simulink model "comVisualization"  (Simulink 8.4)
settings: Solver=FixedStepDiscrete  StartTime=0.0  StopTime=inf  FixedStep=0.010  RelTol=1e-3
InitFcn:
  | Init;
  | visualizerParameters;
values from neighbouring files (symbols this model uses):
  figureHandle = figure    [visualizerParameters.m]
  footLength = 0.15    [visualizerParameters.m]
  footWidth = 0.08    [visualizerParameters.m]
  l_ankle_pitch = 18    [visualizerParameters.m]
  l_ankle_roll = 19    [visualizerParameters.m]
  r_ankle_pitch = 24    [visualizerParameters.m]
  r_ankle_roll = 25    [visualizerParameters.m]
  Ts = 0.006    [Init.m]
libraries: WBCLibrary x9
settings Model: Creator=jorhabib  LastModifiedBy=pucci
settings DataIOCC: SignalLoggingSaveFormat=Dataset
settings OptimizationCC: ExpressionDepthLimit=128
settings DebuggingCC: UnderspecifiedInitializationDetection=Simplified  MergeDetectMultiDrivingBlocksExec=error  FcnCallInpInsideContextMsg=EnableAllAsError  StateNameClashWarn=none
settings GRTTargetCC: CombineOutputUpdateFcns=on  GRTInterface=off

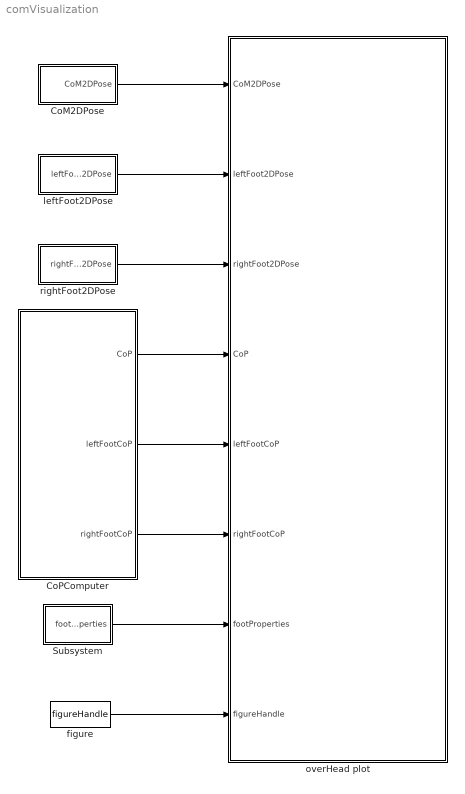
== system comVisualization ==
  CoM2DPose : Subsystem
  CoPComputer : Subsystem
  Subsystem : Subsystem
  figure : Constant  Value=figureHandle
  leftFoot2DPose : Subsystem
  overHead plot : MATLAB Function  TreatAsAtomicUnit=on
  rightFoot2DPose : Subsystem
  wires:
  CoM2DPose/1(CoM2DPose) -> overHead plot/1(CoM2DPose)
  CoPComputer/3(rightFootCoP) -> overHead plot/6(rightFootCoP)
  CoPComputer/2(leftFootCoP) -> overHead plot/5(leftFootCoP)
  CoPComputer/1(CoP) -> overHead plot/4(CoP)
  rightFoot2DPose/1(rightFoot2DPose) -> overHead plot/3(rightFoot2DPose)
  leftFoot2DPose/1(leftFoot2DPose) -> overHead plot/2(leftFoot2DPose)
  figure/1 -> overHead plot/8(figureHandle)
  Subsystem/1(footProperties) -> overHead plot/7(footProperties)

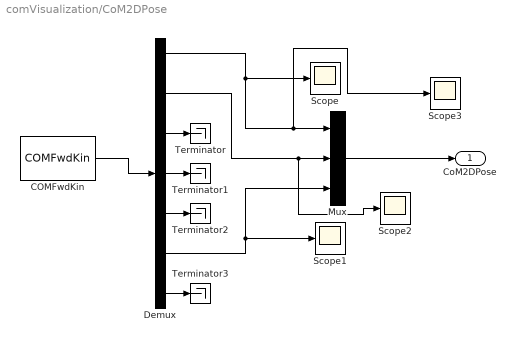
== system comVisualization/CoM2DPose ==
  "COMFwdKin " : WBCLibrary/wholeBodyModel/Forward Kinematics/COMFwdKin   robotName=robotName  localName=localName
  Demux : Demux  Outputs=7
  Mux : Mux  Inputs=3
  Scope{,1..3} (4 alike) : Scope
      Scope1 settings: SaveName=ScopeData5
      Scope2 settings: SaveName=ScopeData6
      Scope3 settings: SaveName=ScopeData7
  Terminator{,1..3} (4 alike) : Terminator
  CoM2DPose : Outport
  wires:
  Demux/3 -> Terminator/1
  Demux/2 -> Scope2/1, Mux/2
  "COMFwdKin "/1 -> Demux/1
  Demux/4 -> Terminator1/1
  Demux/5 -> Terminator2/1
  Mux/1 -> CoM2DPose/1
  Demux/6 -> Mux/3, Scope1/1
  Demux/1 -> Scope/1, Scope3/1, Mux/1
  Demux/7 -> Terminator3/1

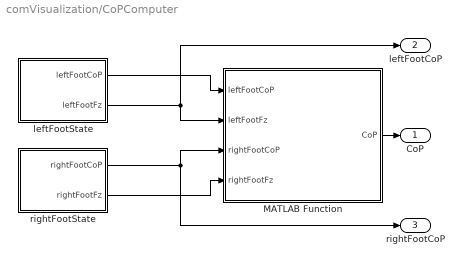
== system comVisualization/CoPComputer ==
  MATLAB Function : MATLAB Function  TreatAsAtomicUnit=on
  leftFootState : Subsystem
  rightFootState : Subsystem
  CoP : Outport
  leftFootCoP : Outport  Port=2
  rightFootCoP : Outport  Port=3
  wires:
  rightFootState/1(rightFootCoP) -> rightFootCoP/1, MATLAB Function/3(rightFootCoP)
  leftFootState/1(leftFootCoP) -> MATLAB Function/1(leftFootCoP)
  leftFootState/2(leftFootFz) -> leftFootCoP/1, MATLAB Function/2(leftFootFz)
  rightFootState/2(rightFootFz) -> MATLAB Function/4(rightFootFz)
  MATLAB Function/1(CoP) -> CoP/1

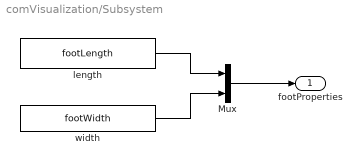
== system comVisualization/Subsystem ==
  Mux : Mux  Inputs=2
  length : Constant  Value=footLength
  width : Constant  Value=footWidth
  footProperties : Outport
  wires:
  length/1 -> Mux/1
  Mux/1 -> footProperties/1
  width/1 -> Mux/2

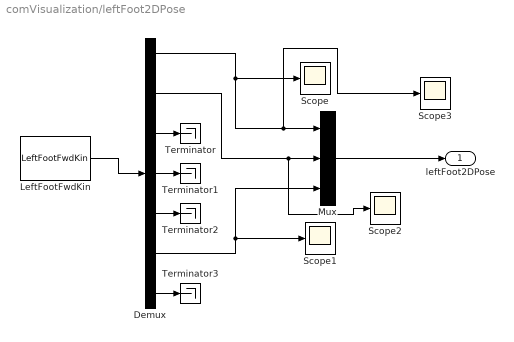
== system comVisualization/leftFoot2DPose ==
  Demux : Demux  Outputs=7
  LeftFootFwdKin : WBCLibrary/wholeBodyModel/Forward Kinematics/LeftFootFwdKin  robotName=robotName  localName=localName
      link override Input Param. for forwardKinematics and  computeJacobians 4: Value=zeros(ROBOT_DOF+6,1)
  Mux : Mux  Inputs=3
  Scope{,1..3} (4 alike) : Scope
      Scope1 settings: SaveName=ScopeData2
      Scope2 settings: SaveName=ScopeData3
      Scope3 settings: SaveName=ScopeData4
  Terminator{,1..3} (4 alike) : Terminator
  leftFoot2DPose : Outport
  wires:
  Demux/3 -> Terminator/1
  Demux/2 -> Scope2/1, Mux/2
  LeftFootFwdKin/1 -> Demux/1
  Demux/4 -> Terminator1/1
  Demux/5 -> Terminator2/1
  Mux/1 -> leftFoot2DPose/1
  Demux/6 -> Mux/3, Scope1/1
  Demux/1 -> Scope/1, Scope3/1, Mux/1
  Demux/7 -> Terminator3/1

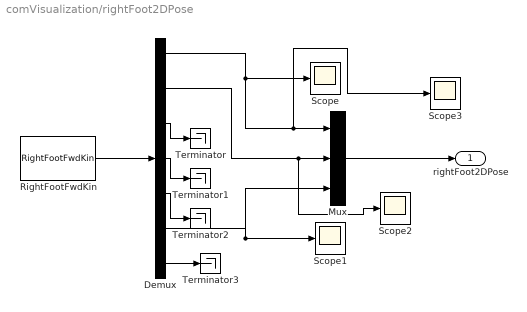
== system comVisualization/rightFoot2DPose ==
  Demux : Demux  Outputs=7
  Mux : Mux  Inputs=3
  RightFootFwdKin : WBCLibrary/wholeBodyModel/Forward Kinematics/RightFootFwdKin  robotName=robotName  localName=localName
  Scope{,1..3} (4 alike) : Scope
      Scope1 settings: SaveName=ScopeData2
      Scope2 settings: SaveName=ScopeData3
      Scope3 settings: SaveName=ScopeData4
  Terminator{,1..3} (4 alike) : Terminator
  rightFoot2DPose : Outport
  wires:
  Demux/3 -> Terminator/1
  Demux/2 -> Scope2/1, Mux/2
  RightFootFwdKin/1 -> Demux/1
  Demux/4 -> Terminator1/1
  Demux/5 -> Terminator2/1
  Mux/1 -> rightFoot2DPose/1
  Demux/6 -> Mux/3, Scope1/1
  Demux/1 -> Scope/1, Scope3/1, Mux/1
  Demux/7 -> Terminator3/1

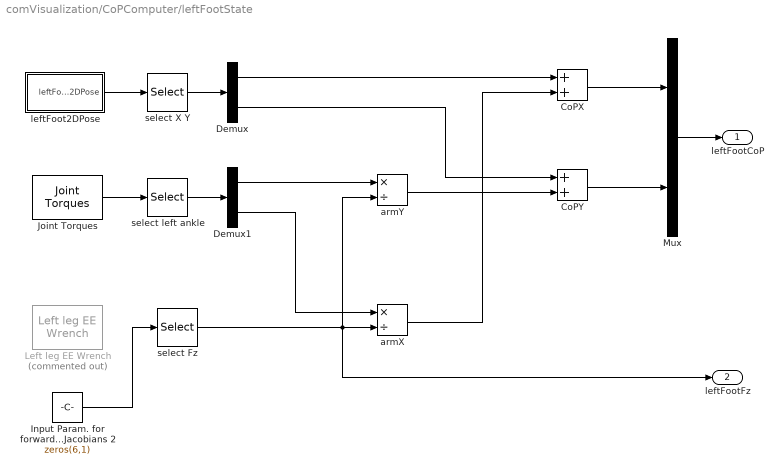
== system comVisualization/CoPComputer/leftFootState ==
  CoPX : Sum
  CoPY : Sum
  Demux : Demux  Outputs=2
  Demux1 : Demux  Outputs=2
  Input Param. for forwardKinematics and  computeJacobians 2 : Constant  Value=zeros(6,1)  OutDataTypeStr=double  SampleTime=Ts
  Joint Torques : WBCLibrary/wholeBodyStates/Joint Torques  robotName=robotName  localName=localName
  Left leg EE Wrench : WBCLibrary/wholeBodyStates/Left leg EE Wrench  Commented=on  robotName=robotName  localName=localName
  Mux : Mux  Inputs=2
  armX : Product  Inputs=*/
  armY : Product  Inputs=*/
  leftFoot2DPose : Subsystem
  select Fz : Selector  InputPortWidth=6  Indices=[3]
  select X Y : Selector  InputPortWidth=3  Indices=[1, 2]
  select left ankle : Selector  InputPortWidth=25  Indices=[l_ankle_pitch, l_ankle_roll]
  leftFootCoP : Outport
  leftFootFz : Outport  Port=2
  wires:
  select left ankle/1 -> Demux1/1
  CoPY/1 -> Mux/2
  CoPX/1 -> Mux/1
  armY/1 -> CoPY/2
  Mux/1 -> leftFootCoP/1
  Demux1/2 -> armX/1
  Demux/2 -> CoPY/1
  Demux/1 -> CoPX/1
  Joint Torques/1 -> select left ankle/1
  armX/1 -> CoPX/2
  Demux1/1 -> armY/1
  select X Y/1 -> Demux/1
  leftFoot2DPose/1(leftFoot2DPose) -> select X Y/1
  select Fz/1 -> leftFootFz/1, armX/2, armY/2
  Input Param. for forwardKinematics and  computeJacobians 2/1 -> select Fz/1

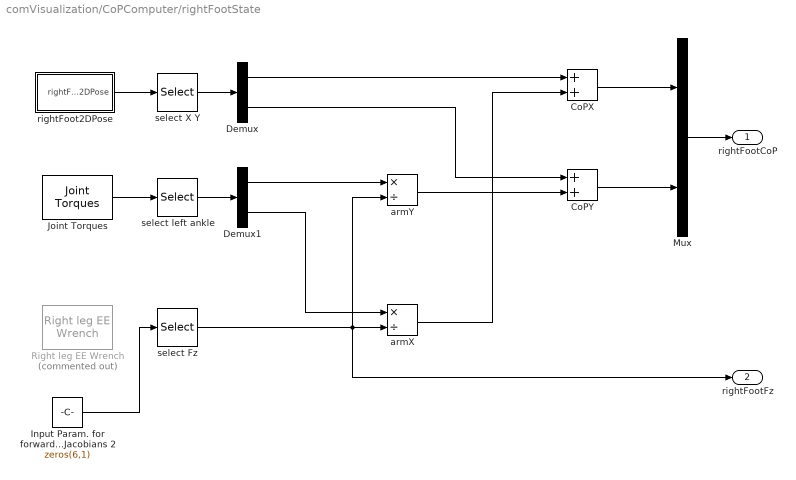
== system comVisualization/CoPComputer/rightFootState ==
  CoPX : Sum
  CoPY : Sum
  Demux : Demux  Outputs=2
  Demux1 : Demux  Outputs=2
  Input Param. for forwardKinematics and  computeJacobians 2 : Constant  Value=zeros(6,1)  OutDataTypeStr=double  SampleTime=Ts
  Joint Torques : WBCLibrary/wholeBodyStates/Joint Torques  robotName=robotName  localName=localName
  Mux : Mux  Inputs=2
  Right leg EE Wrench : WBCLibrary/wholeBodyStates/Right leg EE Wrench  Commented=on  robotName=robotName  localName=localName
  armX : Product  Inputs=*/
  armY : Product  Inputs=*/
  rightFoot2DPose : Subsystem
  select Fz : Selector  InputPortWidth=6  Indices=[3]
  select X Y : Selector  InputPortWidth=3  Indices=[1, 2]
  select left ankle : Selector  InputPortWidth=25  Indices=[r_ankle_pitch, r_ankle_roll]
  rightFootCoP : Outport
  rightFootFz : Outport  Port=2
  wires:
  select left ankle/1 -> Demux1/1
  CoPY/1 -> Mux/2
  CoPX/1 -> Mux/1
  armY/1 -> CoPY/2
  Mux/1 -> rightFootCoP/1
  Demux1/2 -> armX/1
  Demux/2 -> CoPY/1
  Demux/1 -> CoPX/1
  Joint Torques/1 -> select left ankle/1
  armX/1 -> CoPX/2
  Demux1/1 -> armY/1
  select X Y/1 -> Demux/1
  rightFoot2DPose/1(rightFoot2DPose) -> select X Y/1
  select Fz/1 -> rightFootFz/1, armX/2, armY/2
  Input Param. for forwardKinematics and  computeJacobians 2/1 -> select Fz/1

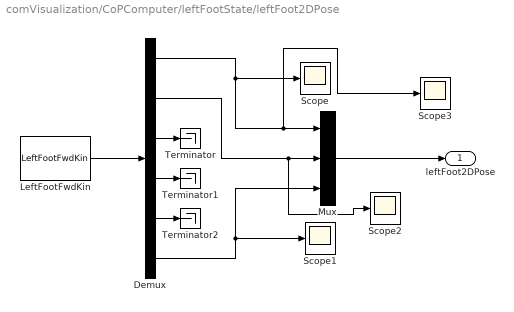
== system comVisualization/CoPComputer/leftFootState/leftFoot2DPose ==
  Demux : Demux  Outputs=6
  LeftFootFwdKin : WBCLibrary/wholeBodyModel/Forward Kinematics/LeftFootFwdKin  robotName=robotName  localName=localName
      link override Input Param. for forwardKinematics and  computeJacobians 4: Value=zeros(ROBOT_DOF+6,1)
  Mux : Mux  Inputs=3
  Scope{,1..3} (4 alike) : Scope
      Scope1 settings: SaveName=ScopeData2
      Scope2 settings: SaveName=ScopeData3
      Scope3 settings: SaveName=ScopeData4
  Terminator : Terminator
  Terminator1 : Terminator
  Terminator2 : Terminator
  leftFoot2DPose : Outport
  wires:
  Demux/3 -> Terminator/1
  Demux/2 -> Scope2/1, Mux/2
  LeftFootFwdKin/1 -> Demux/1
  Demux/4 -> Terminator1/1
  Demux/5 -> Terminator2/1
  Mux/1 -> leftFoot2DPose/1
  Demux/6 -> Mux/3, Scope1/1
  Demux/1 -> Scope/1, Scope3/1, Mux/1

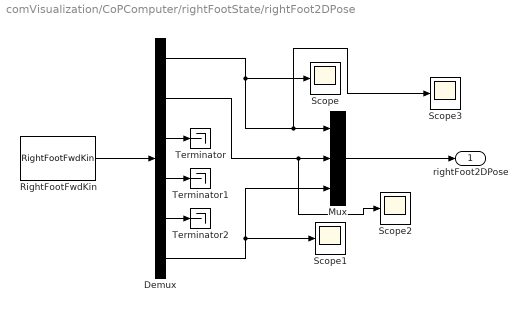
== system comVisualization/CoPComputer/rightFootState/rightFoot2DPose ==
  Demux : Demux  Outputs=6
  Mux : Mux  Inputs=3
  RightFootFwdKin : WBCLibrary/wholeBodyModel/Forward Kinematics/RightFootFwdKin  robotName=robotName  localName=localName
  Scope{,1..3} (4 alike) : Scope
      Scope1 settings: SaveName=ScopeData2
      Scope2 settings: SaveName=ScopeData3
      Scope3 settings: SaveName=ScopeData4
  Terminator : Terminator
  Terminator1 : Terminator
  Terminator2 : Terminator
  rightFoot2DPose : Outport
  wires:
  Demux/3 -> Terminator/1
  Demux/2 -> Scope2/1, Mux/2
  RightFootFwdKin/1 -> Demux/1
  Demux/4 -> Terminator1/1
  Demux/5 -> Terminator2/1
  Mux/1 -> rightFoot2DPose/1
  Demux/6 -> Mux/3, Scope1/1
  Demux/1 -> Scope/1, Scope3/1, Mux/1

== matlab function CoPComputer/MATLAB Function ==
  data: leftFootCoP input double; leftFootFz input double; CoP output double; rightFootCoP input double; rightFootFz input double
function CoP = fcn(leftFootCoP, leftFootFz, rightFootCoP, rightFootFz)
leftFootCoPX = leftFootCoP(1);
leftFootCoPY = leftFootCoP(2);
rightFootCoPX = rightFootCoP(1);
rightFootCoPY = rightFootCoP(2);
totFz = leftFootFz + rightFootFz;

CoPX = (leftFootCoPX * leftFootFz + rightFootCoPX * rightFootFz) / totFz; 
CoPY = (leftFootCoPY * leftFootFz + rightFootCoPY * rightFootFz) / totFz;

CoP = [CoPX, CoPY];

== matlab function overHead plot ==
  data: CoM2DPose input double; leftFoot2DPose input double; rightFoot2DPose input double; CoP input double; leftFootCoP input double; rightFootCoP input double; footProperties input double; figureHandle input double
function fcn(CoM2DPose, leftFoot2DPose, rightFoot2DPose, CoP, leftFootCoP, rightFootCoP, footProperties, figureHandle)
% constants
LEFT_FOOT_COLOR = 'r';
RIGHT_FOOT_COLOR = 'g';
CoM_COLOR = 'k';
CoP_COLOR = 'b';
FOOT_SCALE_FACTOR = 3;
CIRCLE_RADIUS = 4;

footLength = footProperties(1);
footWidth = footProperties(2);

leftFootCentroid = [leftFoot2DPose(1), leftFoot2DPose(2)];
leftFootYaw = 0.0; %leftFoot2DPose(3);
[leftX, leftY] = computeFourFootPolygonVertices(leftFootCentroid, leftFootYaw, footLength, footWidth);

rightFootCentroid = [rightFoot2DPose(1), rightFoot2DPose(2)];
rightFootYaw = 0.0; %rightFoot2DPose(3);
[rightX, rightY] = computeFourFootPolygonVertices(rightFootCentroid, rightFootYaw, footLength, footWidth);

prepareFigure(figureHandle, CoM2DPose, footLength, FOOT_SCALE_FACTOR);
drawCircle(CoM2DPose, CIRCLE_RADIUS, CoM_COLOR, figureHandle)
plotFootPolygon(leftX, leftY, LEFT_FOOT_COLOR, figureHandle);
plotFootPolygon(rightX, rightY, RIGHT_FOOT_COLOR, figureHandle);

function [x, y] = computeFourFootPolygonVertices(centroid, footYaw, footLength, footWidth)
NUMBER_OF_VERTICES = 4;

centroidX = centroid(1);
centroidY = centroid(2);
halfFootLength = footLength/2;
halfFootWidth = footWidth/2;
x = zeros(NUMBER_OF_VERTICES);
y = zeros(NUMBER_OF_VERTICES);

tempX = centroidX + halfFootLength;
tempY = centroidY + halfFootWidth;
[rotX, rotY] = rotate2DVector(tempX, tempY, footYaw);
x(1) = rotX;
y(1) = rotY;

tempX = centroidX - halfFootLength;
tempY = centroidY + halfFootWidth;
[rotX, rotY] = rotate2DVector(tempX, tempY, footYaw);
x(2) = rotX;
y(2) = rotY;

tempX = centroidX - halfFootLength;
tempY = centroidY - halfFootWidth;
[rotX, rotY] = rotate2DVector(tempX, tempY, footYaw);
x(3) = rotX;
y(3) = rotY;

tempX = centroidX + halfFootLength;
tempY = centroidY - halfFootWidth;
[rotX, rotY] = rotate2DVector(tempX, tempY, footYaw);
x(4) = rotX;
y(4) = rotY;

function plotFootPolygon(x, y, color, figureHandle)
numberOfVertices = length(x);

for i = 1 : numberOfVertices
    if i < numberOfVertices
        drawLine([x(i),y(i)],[x(i+1), y(i+1)], color, figureHandle);
    else
        drawLine([x(i),y(i)],[x(1), y(1)], color, figureHandle);
    end
end

function [] = drawLine(p1, p2, color, figureHandle)
theta = atan2( p2(2) - p1(2), p2(1) - p1(1));
r = sqrt( (p2(1) - p1(1))^2 + (p2(2) - p1(2))^2);

line = linspace(0,r,10);
x = p1(1) + line*cos(theta);
y = p1(2) + line*sin(theta);

figure(figureHandle);
plot(x, y, color)
drawnow;
hold on

function [] = drawCircle(position, radius, color, figureHandle)
x = position(1);
y = position(2);

figure(figureHandle);
plot(x, y, 'Color', color, 'Marker', 'o', 'MarkerSize', radius)
drawnow;
hold on

function [newX,newY] = rotate2DVector(x, y, angle)
newX = x * cos(angle) - y * sin(angle);
newY = x * sin(angle) + y * cos(angle);

function [] = prepareFigure(figureHandle, CoM2DPose, footLength, factor)
addendum = factor * footLength;
CoM2DPoseX = CoM2DPose(1);
CoM2DPoseY = CoM2DPose(2);

xmax = CoM2DPoseX + addendum;
xmin = CoM2DPoseX - addendum;
ymax = CoM2DPoseY + addendum;
ymin = CoM2DPoseY - addendum;

clf(figureHandle);
axis([xmin xmax ymin ymax])
hold on;
